simulink model "Regulator_Flow_Sim_1"  (R2022b)
settings: Solver=VariableStepAuto  StartTime=0.0  StopTime=6  RelTol=1e-3
values from neighbouring files (symbols this model uses):
  A_3 = 60*1e-6    (= 6e-05)    [Init_Regulator_Flow_Sim.m]
  Cd_3 = 0.7    [Init_Regulator_Flow_Sim.m]
  Feedforward = 25    [Init_Regulator_Flow_Sim.m]
  gamma_N2 = 1.4    [Init_Regulator_Flow_Sim.m]
  K_v_4 = 0.5    [Init_Regulator_Flow_Sim.m]
  Kv_1_max = 1    [Init_Regulator_Flow_Sim.m]
  Kv_2 = 1    [Init_Regulator_Flow_Sim.m]
  m_1_0 = V_1*rho_1_0    (= 2.59009009009)    [Init_Regulator_Flow_Sim.m]
  m_2_0 = rho_2_0*(V_2-(m_3_0/rho_L))    (= 0.225225225225)    [Init_Regulator_Flow_Sim.m]
  m_3_0 = 8    [Init_Regulator_Flow_Sim.m]
  P_2_0 = P_2_0*1e5    (= 4000000)    [Init_Regulator_Flow_Sim.m]
  P_atm = 0    [Init_Regulator_Flow_Sim.m]
  Pst = 101325    [Init_Regulator_Flow_Sim.m]
  R_N2 = 296    [Init_Regulator_Flow_Sim.m]
  rho_1_0 = (P_1_0)/(R_N2*T_0_N2)    (= 259.009009009)    [Init_Regulator_Flow_Sim.m]
  rho_L = 1000    [Init_Regulator_Flow_Sim.m]
  rhost = Pst/(R_N2*Tst)    (= 1.25320955222)    [Init_Regulator_Flow_Sim.m]
  T_0_N2 = 300    [Init_Regulator_Flow_Sim.m]
  Tst = 273.15    [Init_Regulator_Flow_Sim.m]
  V_1 = V_1*1e-3    (= 0.01)    [Init_Regulator_Flow_Sim.m]
  V_2 = V_2*1e-3    (= 0.013)    [Init_Regulator_Flow_Sim.m]
libraries: slpidlib x2
settings Model: Creator=marti  LastModifiedBy=marti

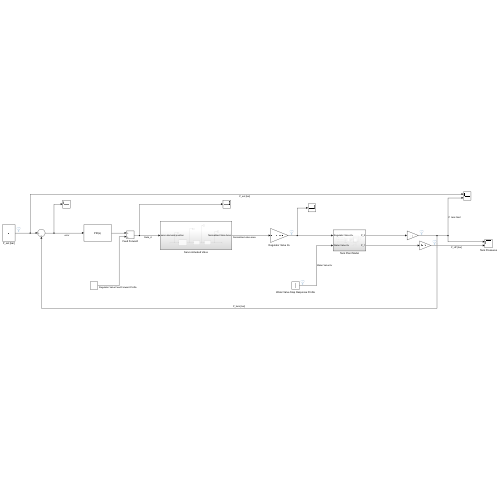
[thumbnail: Simulink's stored preview of the top-level diagram]
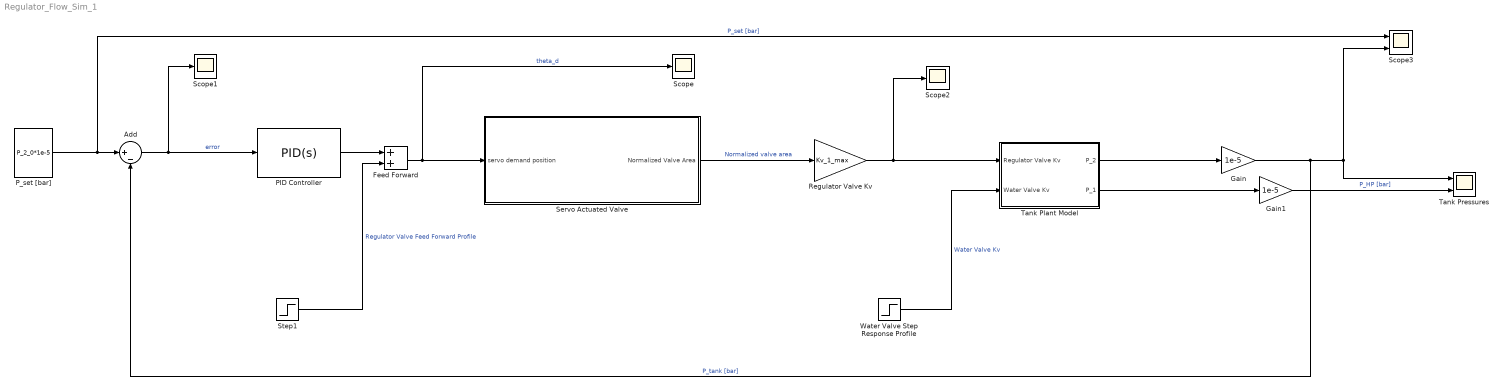
== system Regulator_Flow_Sim_1 ==
  Add : Sum  Inputs=|+-
  Feed Forward : Sum
  Gain : Gain  Gain=1e-5
  Gain1 : Gain  Gain=1e-5
  PID Controller : slpidlib/PID Controller  Controller=PID  Form=Parallel  TimeDomain=Continuous-time  UseExternalTs=off  SampleTime=-1  IntegratorMethod=Forward Euler  FilterMethod=Forward Euler  ControllerParametersSource=internal  P=1.5  I=3  UseKiTs=off  D=0  N=100  UseFilter=on  TunerSelectOption=Transfer Function Based (PID Tuner App)  InitialConditionSource=internal  InitialConditionForIntegrator=0  InitialConditionForFilter=0  DifferentiatorICPrevScaledInput=0  ExternalReset=none  TrackingMode=off  Kt=1  LimitOutput=off  SatLimitsSource=internal  UpperSaturationLimit=180  LowerSaturationLimit=0  LinearizeAsGain=on  AntiWindupMode=clamping  Kb=1  LimitIntegrator=on  UpperIntegratorSaturationLimit=20  LowerIntegratorSaturationLimit=-20  POutMin=[]  POutMax=[]  IOutMin=[]  IOutMax=[]  DOutMin=[]  DOutMax=[]  NOutMin=[]  NOutMax=[]  SumOutMin=[]  SumOutMax=[]  SaturationOutMin=[]  SaturationOutMax=[]  PParamMin=[]  PParamMax=[]  IParamMin=[]  IParamMax=[]  DParamMin=[]  DParamMax=[]  NParamMin=[]  NParamMax=[]  KbParamMin=[]  KbParamMax=[]  KtParamMin=[]  KtParamMax=[]  KbOutMin=[]  KbOutMax=[]  KtOutMin=[]  KtOutMax=[]  IntegratorOutMin=[]  IntegratorOutMax=[]  FilterOutMin=[]  FilterOutMax=[]  SumI1OutMin=[]  SumI1OutMax=[]  SumI2OutMin=[]  SumI2OutMax=[]  SumI3OutMin=[]  SumI3OutMax=[]  SumI4OutMin=[]  SumI4OutMax=[]  SumDOutMin=[]  SumDOutMax=[]  DifferentiatorOutMin=[]  DifferentiatorOutMax=[]  FilterDiffOutCoefMin=[]  FilterDiffOutCoefMax=[]  ReciprocalOutMin=[]  ReciprocalOutMax=[]  SumDenOutMin=[]  SumDenOutMax=[]  SumNumOutMin=[]  SumNumOutMax=[]  DivideOutMin=[]  DivideOutMax=[]  UdiffTsProdOutMin=[]  UdiffTsProdOutMax=[]  NTsProdOutMin=[]  NTsProdOutMax=[]  UintegralTsProdOutMin=[]  UintegralTsProdOutMax=[]  UngainTsProdOutMin=[]  UngainTsProdOutMax=[]  ClampingZeroOutDataTypeStr=Inherit: Inherit via back propagation  ClampingZeroOutMin=[]  ClampingZeroOutMax=[]  FilterDenConstantOutDataTypeStr=Inherit: Inherit via back propagation  FilterDenConstantOutMin=[]  FilterDenConstantOutMax=[]  PCopyOutDataTypeStr=Inherit: Inherit via back propagation  PCopyOutMin=[]  PCopyOutMax=[]  NCopyOutDataTypeStr=Inherit: Inherit via back propagation  NCopyOutMin=[]  NCopyOutMax=[]  IntegratorContinuousStateAttributes=''  IntegratorStateMustResolveToSignalObject=off  IntegratorRTWStateStorageClass=Auto  FilterContinuousStateAttributes=''  FilterStateMustResolveToSignalObject=off  FilterRTWStateStorageClass=Auto  ParallelPVariant=InternalParameters  IdealPVariant=Disabled  IVariant=InternalParameters  DVariant=InternalParameters  IntegratorVariant=Continuous  SatVariant=Disabled  AWVariant=Passthrough  PCopyVariant=Disabled  TRVariant=Disabled  FdbkBlocksVariant=Forward  IdealPFdbkVariant=Disabled  SatFdbkVariant=Disabled  DerivativeFilterVariant=ContFilter  NVariant=InternalParameters  NCopyVariant=Disabled  FilterICVariant=InternalICsFilter  IntegratorICVariant=InternalICs  ExternalResetVariant=Disabled  TRSumVariant=Passthrough  SumFdbkVariant=Disabled  SumVariant=Sum_PID  TsampFilterVariant=InternalTs  TsampNgainVariant=Passthrough  TsampIntegralVariant=Passthrough  ExternalSaturationOutDataTypeStr=Inherit: Same as second input
  P_set [bar] : Constant  Value=P_2_0*1e-5
  Regulator Valve Kv : Gain  Gain=Kv_1_max
  Scope : Scope
  Scope1 : Scope
  Scope2 : Scope
  Scope3 : Scope  NumInputPorts=2
  Servo Actuated Valve : Subsystem
  Step1 : Step  After=Feedforward  SampleTime=0
  Tank Plant Model : Subsystem
  Tank Pressures : Scope  NumInputPorts=2
  Water Valve Step Response Profile : Step  After=Kv_2  SampleTime=0
  wires:
  Water Valve Step Response Profile/1 -> Tank Plant Model/2(Water Valve Kv)  "Water Valve Kv"
  Tank Plant Model/1(P_2) -> Gain/1
  Tank Plant Model/2(P_1) -> Gain1/1
  Servo Actuated Valve/1(Normalized Valve Area) -> Regulator Valve Kv/1  "Normalized valve area"
  Feed Forward/1 -> Scope/1, Servo Actuated Valve/1(servo demand position)  "theta_d"
  Add/1 -> Scope1/1, PID Controller/1  "error"
  Gain/1 -> Scope3/2, Tank Pressures/1, Add/2  "P_tank [bar]"
  Gain1/1 -> Tank Pressures/2  "P_HP [bar]"
  Regulator Valve Kv/1 -> Scope2/1, Tank Plant Model/1(Regulator Valve Kv)
  P_set [bar]/1 -> Scope3/1, Add/1  "P_set [bar]"
  PID Controller/1 -> Feed Forward/1
  Step1/1 -> Feed Forward/2  "Regulator Valve Feed Forward Profile"

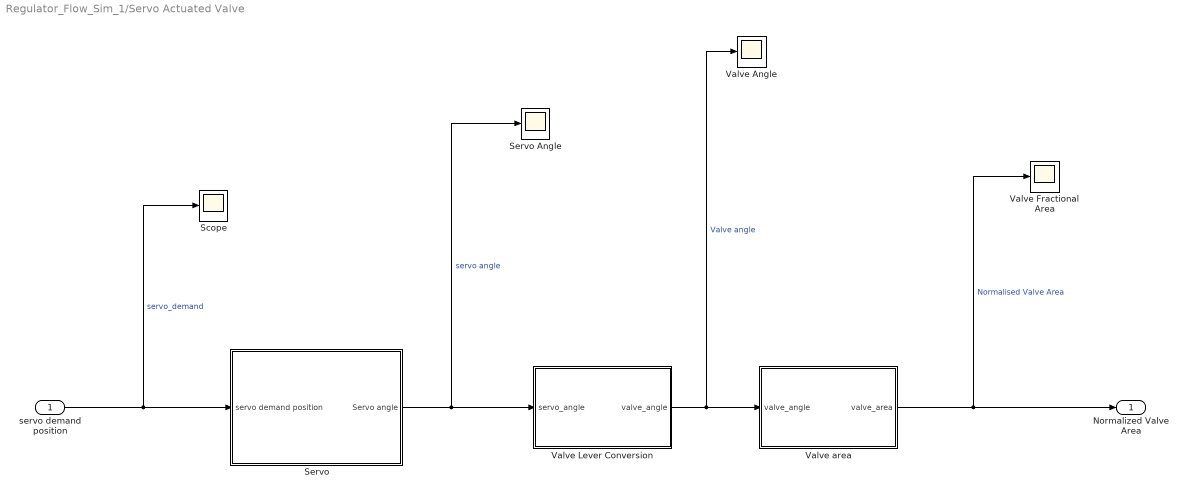
== system Regulator_Flow_Sim_1/Servo Actuated Valve ==
  servo demand position : Inport
  " Valve Lever Conversion" : MATLAB Function  TreatAsAtomicUnit=on
  " Valve area" : MATLAB Function  TreatAsAtomicUnit=on
  Scope : Scope
  Servo : Subsystem
  Servo Angle : Scope
  Valve Angle : Scope
  Valve Fractional Area : Scope
  Normalized Valve Area : Outport
  wires:
  " Valve area"/1(valve_area) -> Normalized Valve Area/1, Valve Fractional Area/1  "Normalised Valve Area"
  " Valve Lever Conversion"/1(valve_angle) -> " Valve area"/1(valve_angle), Valve Angle/1  "Valve angle"
  servo demand position/1 -> Scope/1, Servo/1(servo demand position)  "servo_demand"
  Servo/1(Servo angle) -> " Valve Lever Conversion"/1(servo_angle), Servo Angle/1  "servo angle"

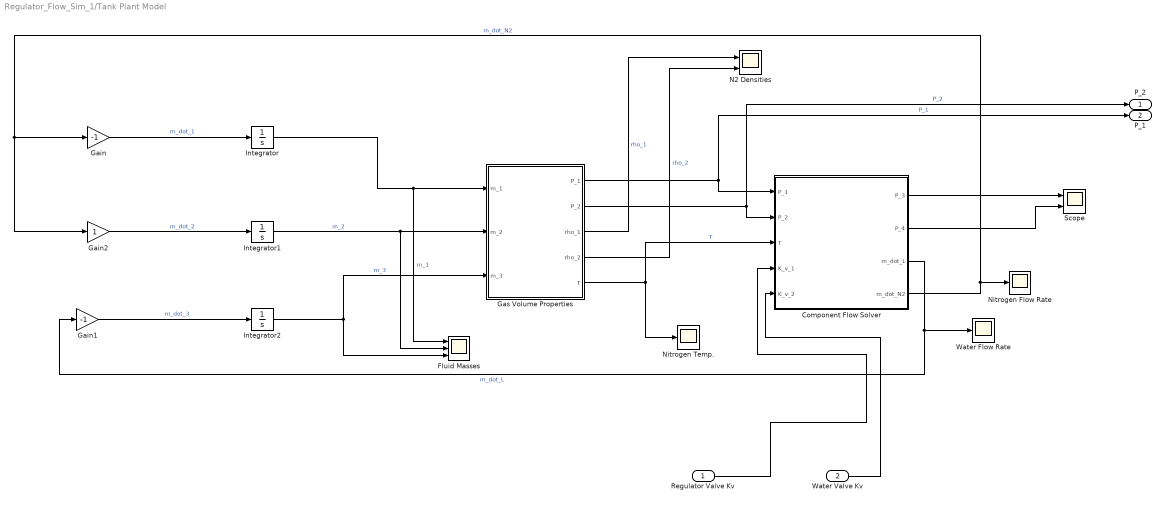
== system Regulator_Flow_Sim_1/Tank Plant Model ==
  Regulator Valve Kv : Inport
  Water Valve Kv : Inport  Port=2
  Component Flow Solver : MATLAB Function  TreatAsAtomicUnit=on
  Fluid Masses : Scope  NumInputPorts=3
  Gain : Gain  Gain=-1
  Gain1 : Gain  Gain=-1
  Gain2 : Gain
  Gas Volume Properties : MATLAB Function  TreatAsAtomicUnit=on
  Integrator : Integrator  InitialCondition=m_1_0
  Integrator1 : Integrator  InitialCondition=m_2_0
  Integrator2 : Integrator  InitialCondition=m_3_0
  N2 Densities : Scope  NumInputPorts=2
  Nitrogen Flow Rate : Scope
  Nitrogen Temp. : Scope
  Scope : Scope  NumInputPorts=2
  Water Flow Rate : Scope
  P_2 : Outport
  P_1 : Outport  Port=2
  wires:
  Gas Volume Properties/1(P_1) -> P_1/1, Component Flow Solver/1(P_1)  "P_1"
  Gain/1 -> Integrator/1  "m_dot_1"
  Component Flow Solver/1(P_3) -> Scope/1
  Integrator1/1 -> Fluid Masses/2, Gas Volume Properties/2(m_2)  "m_2"
  Integrator/1 -> Fluid Masses/1, Gas Volume Properties/1(m_1)  "m_1"
  Component Flow Solver/2(P_4) -> Scope/2
  Gain1/1 -> Integrator2/1  "m_dot_3"
  Component Flow Solver/4(m_dot_N2) -> Nitrogen Flow Rate/1, Gain2/1, Gain/1  "m_dot_N2"
  Gain2/1 -> Integrator1/1  "m_dot_2"
  Integrator2/1 -> Gas Volume Properties/3(m_3), Fluid Masses/3  "m_3"
  Gas Volume Properties/2(P_2) -> P_2/1, Component Flow Solver/2(P_2)  "P_2"
  Component Flow Solver/3(m_dot_L) -> Water Flow Rate/1, Gain1/1  "m_dot_L"
  Gas Volume Properties/4(rho_2) -> N2 Densities/2  "rho_2"
  Gas Volume Properties/3(rho_1) -> N2 Densities/1  "rho_1"
  Gas Volume Properties/5(T) -> Nitrogen Temp./1, Component Flow Solver/3(T)  "T"
  Water Valve Kv/1 -> Component Flow Solver/5(K_v_2)
  Regulator Valve Kv/1 -> Component Flow Solver/4(K_v_1)

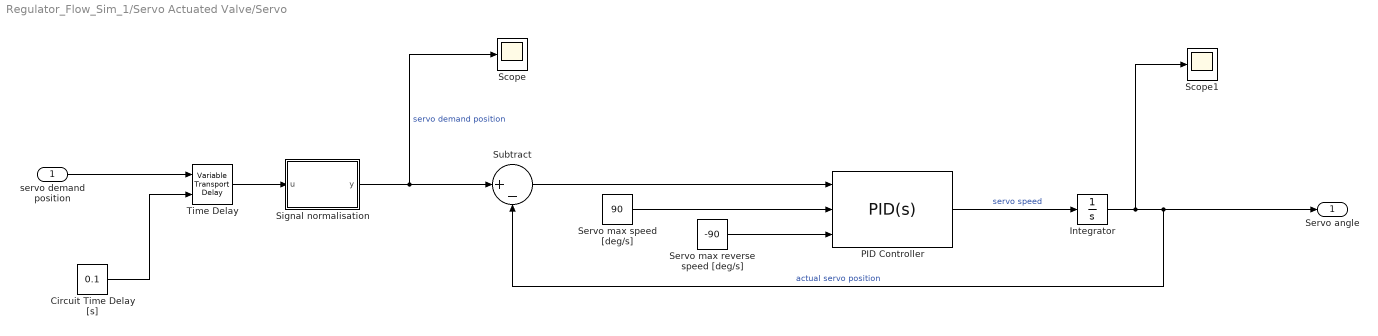
== system Regulator_Flow_Sim_1/Servo Actuated Valve/Servo ==
  servo demand position : Inport
  Circuit Time Delay [s] : Constant  Value=0.1
  Integrator : Integrator
  PID Controller : slpidlib/PID Controller  Controller=PID  Form=Parallel  TimeDomain=Continuous-time  UseExternalTs=off  SampleTime=-1  IntegratorMethod=Forward Euler  FilterMethod=Forward Euler  ControllerParametersSource=internal  P=10  I=1  UseKiTs=off  D=0  N=100  UseFilter=on  TunerSelectOption=Transfer Function Based (PID Tuner App)  InitialConditionSource=internal  InitialConditionForIntegrator=0  InitialConditionForFilter=0  DifferentiatorICPrevScaledInput=0  ExternalReset=none  TrackingMode=off  Kt=1  LimitOutput=on  SatLimitsSource=external  UpperSaturationLimit=inf  LowerSaturationLimit=-inf  LinearizeAsGain=on  AntiWindupMode=none  Kb=1  LimitIntegrator=off  UpperIntegratorSaturationLimit=inf  LowerIntegratorSaturationLimit=-inf  POutMin=[]  POutMax=[]  IOutMin=[]  IOutMax=[]  DOutMin=[]  DOutMax=[]  NOutMin=[]  NOutMax=[]  SumOutMin=[]  SumOutMax=[]  SaturationOutMin=[]  SaturationOutMax=[]  PParamMin=[]  PParamMax=[]  IParamMin=[]  IParamMax=[]  DParamMin=[]  DParamMax=[]  NParamMin=[]  NParamMax=[]  KbParamMin=[]  KbParamMax=[]  KtParamMin=[]  KtParamMax=[]  KbOutMin=[]  KbOutMax=[]  KtOutMin=[]  KtOutMax=[]  IntegratorOutMin=[]  IntegratorOutMax=[]  FilterOutMin=[]  FilterOutMax=[]  SumI1OutMin=[]  SumI1OutMax=[]  SumI2OutMin=[]  SumI2OutMax=[]  SumI3OutMin=[]  SumI3OutMax=[]  SumI4OutMin=[]  SumI4OutMax=[]  SumDOutMin=[]  SumDOutMax=[]  DifferentiatorOutMin=[]  DifferentiatorOutMax=[]  FilterDiffOutCoefMin=[]  FilterDiffOutCoefMax=[]  ReciprocalOutMin=[]  ReciprocalOutMax=[]  SumDenOutMin=[]  SumDenOutMax=[]  SumNumOutMin=[]  SumNumOutMax=[]  DivideOutMin=[]  DivideOutMax=[]  UdiffTsProdOutMin=[]  UdiffTsProdOutMax=[]  NTsProdOutMin=[]  NTsProdOutMax=[]  UintegralTsProdOutMin=[]  UintegralTsProdOutMax=[]  UngainTsProdOutMin=[]  UngainTsProdOutMax=[]  ClampingZeroOutDataTypeStr=Inherit: Inherit via back propagation  ClampingZeroOutMin=[]  ClampingZeroOutMax=[]  FilterDenConstantOutDataTypeStr=Inherit: Inherit via back propagation  FilterDenConstantOutMin=[]  FilterDenConstantOutMax=[]  PCopyOutDataTypeStr=Inherit: Inherit via back propagation  PCopyOutMin=[]  PCopyOutMax=[]  NCopyOutDataTypeStr=Inherit: Inherit via back propagation  NCopyOutMin=[]  NCopyOutMax=[]  IntegratorContinuousStateAttributes=''  IntegratorStateMustResolveToSignalObject=off  IntegratorRTWStateStorageClass=Auto  FilterContinuousStateAttributes=''  FilterStateMustResolveToSignalObject=off  FilterRTWStateStorageClass=Auto  ParallelPVariant=InternalParameters  IdealPVariant=Disabled  IVariant=InternalParameters  DVariant=InternalParameters  IntegratorVariant=Continuous  SatVariant=External  AWVariant=Passthrough  PCopyVariant=Disabled  TRVariant=Disabled  FdbkBlocksVariant=Forward  IdealPFdbkVariant=Disabled  SatFdbkVariant=Disabled  DerivativeFilterVariant=ContFilter  NVariant=InternalParameters  NCopyVariant=Disabled  FilterICVariant=InternalICsFilter  IntegratorICVariant=InternalICs  ExternalResetVariant=Disabled  TRSumVariant=Passthrough  SumFdbkVariant=Disabled  SumVariant=Sum_PID  TsampFilterVariant=InternalTs  TsampNgainVariant=Passthrough  TsampIntegralVariant=Passthrough  ExternalSaturationOutDataTypeStr=Inherit: Same as second input
  Scope : Scope
  Scope1 : Scope
  Servo max reverse speed [deg/s] : Constant  Value=-90
  Servo max speed [deg/s] : Constant  Value=90
  Signal normalisation : MATLAB Function  TreatAsAtomicUnit=on
  Subtract : Sum  Inputs=|+-
  Time Delay : VariableTransportDelay  MaximumDelay=10
  Servo angle : Outport
  wires:
  Servo max reverse speed [deg/s]/1 -> PID Controller/3
  Servo max speed [deg/s]/1 -> PID Controller/2
  PID Controller/1 -> Integrator/1  "servo speed"
  Integrator/1 -> Scope1/1, Servo angle/1, Subtract/2  "actual servo position"
  Subtract/1 -> PID Controller/1
  Signal normalisation/1(y) -> Scope/1, Subtract/1  "servo demand position"
  servo demand position/1 -> Time Delay/1
  Time Delay/1 -> Signal normalisation/1(u)
  Circuit Time Delay [s]/1 -> Time Delay/2

== matlab function Regulator_Flow_Sim_1/Tank Plant Model/Component Flow Solver ==
  data: P_1 input; P_2 input; P_3 output; T input; P_4 output; m_dot_L output; m_dot_N2 output; K_v_1 input; K_v_2 input; Cd_3 parameter; K_v_4 parameter; rho_L parameter; R_N2 parameter; Tst parameter; rhost parameter; P_atm parameter; A_3 parameter; Pst parameter
function [P_3,P_4,m_dot_L,m_dot_N2]= fcn(P_1,P_2,T,K_v_1,K_v_2,Cd_3,K_v_4,rho_L,R_N2,Tst,rhost,P_atm,A_3, Pst)

P_1 = P_1*1e-5;
P_2 = P_2*1e-5;

fun = @(x)paramfun(x,P_1,P_2,T,K_v_1,K_v_2,A_3,Cd_3,K_v_4,rho_L,R_N2,Pst,Tst,rhost,P_atm); %Define set of non-linear equations to rootfind on
x0 = [1,1,1,1]; %Define initial guesses
options = optimoptions('fsolve','Algorithm','levenberg-marquardt');
x = fsolve(fun,x0,options); %Solve system of equations 

P_3 = x(1)*1e5;
P_4 = x(2)*1e5;
m_dot_L = x(3);
m_dot_N2 = x(4);

function F = paramfun(x,P_1,P_2,T,K_v_1,K_v_2,A_3,Cd_3,K_v_4,rho_L,R_N2,Pst,Tst,rhost,P_atm)
P_3 = x(1);
P_4 = x(2);
m_dot_L = x(3);
m_dot_N2 = x(4);

%Regulator Valve
if (P_4 >= 0.528*P_1)
    %non-choked flow
    Q_N = K_v_1*514*(((P_1-P_4)*P_4)/(rhost*T))/sqrt(abs(((P_1-P_4)*P_4)/(rhost*T)));
else
    %choked flow
    Q_N = K_v_1*257*P_1/sqrt(abs(rhost*T));
end
m_dot_c = Q_N*(Pst/(R_N2*Tst))*(1/3600); %Convert standard flow rate to mass flow rate

%Check Valve (K_v_4)
if (P_2 >= 0.528*P_4)
    %non-choked flow
    Q_N = K_v_4*514*(((P_4-P_2)*P_2)/(rhost*T))/sqrt(abs(((P_4-P_2)*P_2)/(rhost*T)));
else
    %choked flow
    Q_N = K_v_4*257*P_4/sqrt(abs(rhost*T));
end
m_dot_d = Q_N*(Pst/(R_N2*Tst))*(1/3600); %Convert standard flow rate to mass flow rate

%Water Control Valve
SG = rho_L/1000; %Calculate specific gravity of propellant (value for water is 1)
Q = K_v_2*((P_2 - P_3)/SG)/sqrt(abs((P_2 - P_3)/SG)); %Calculate volumetric flow rate based on Kv
m_dot_a = Q*rho_L*(1/3600); %Convert standard flow rate to mass flow rate

%Water Orifice
m_dot_b = Cd_3*A_3*2*rho_L*(P_3*1e5 - P_atm)/sqrt(abs(2*rho_L*(P_3*1e5 - P_atm)));

F = [m_dot_L - m_dot_a, m_dot_L - m_dot_b, m_dot_N2 - m_dot_c, m_dot_N2 - m_dot_d];

== matlab function Regulator_Flow_Sim_1/Tank Plant Model/Gas Volume Properties ==
  data: P_1 output; P_2 output; m_1 input; rho_1 output; m_2 input; m_3 input; rho_2 output; T output; V_1 parameter; V_2 parameter; T_0_N2 parameter; rho_1_0 parameter; gamma_N2 parameter; R_N2 parameter; rho_L parameter
function [P_1, P_2, rho_1, rho_2, T]= fcn(m_1, m_2, m_3, V_1, V_2, T_0_N2, rho_1_0, gamma_N2, R_N2, rho_L)

rho_1 = m_1/V_1; %Find the HP tank gas density
rho_2 = m_2/(V_2 - m_3/rho_L); %Find the ullage gas density
T = T_0_N2*(rho_1/rho_1_0)^(gamma_N2 - 1); %Find the ullage gas temperature (assumiong adiabatic expansion)
P_1 = rho_1*R_N2*T; %Find the HP gas pressure
P_2 = rho_2*R_N2*T; %Find the ullage gas pressure (Tank pressure)

== matlab function Regulator_Flow_Sim_1/Servo Actuated Valve/ Valve Lever Conversion ==
  data: servo_angle input; valve_angle output
function valve_angle = fcn(servo_angle)

theta = deg2rad(servo_angle - 20);

% Define lengths of the different levers
g = 42; %Distance between pivots [mm]
a = 20; %Servo Horn Length [mm]
b = 38; %Valve Lever Length [mm]
h = 61; %Connecting linkage length [mm]

fun = @(x)paramfun(x,theta,g,a,b,h); %Define set of non-linear equations to rootfind on
x0 = [pi/2,pi]; %Define initial guesses
options = optimoptions('fsolve','Algorithm','levenberg-marquardt');
x = fsolve(fun,x0,options); %Solve system of equations 

psi = x(2);

valve_angle = rad2deg(psi) - 66;

% Function used for iteratively solving the 
function F = paramfun(x, theta,g,a,b,h)
phi = x(1);
psi = x(2);
F = [a*cos(theta) - h*cos(phi) - b*cos(psi) + g, a*sin(theta) + h*sin(phi) - b*sin(psi)];

== matlab function Regulator_Flow_Sim_1/Servo Actuated Valve/ Valve area ==
  data: valve_angle input; valve_area output
function valve_area = fcn(valve_angle)
valve_angle = valve_angle - 5; %Account for first part of rotation where valve doesn't open at all
if valve_angle < 0
    valve_area = 0;
else
    valve_area = 1.1*((5*10^-6)*valve_angle^3 - 0.0006*valve_angle^2 + 0.0278*valve_angle); %calculate normalised valve area
end

== matlab function Regulator_Flow_Sim_1/Servo Actuated Valve/Servo/Signal normalisation ==
  data: u input; y output
function y = fcn(u)
if u < 0
    y = 0;
else 
    if u > 180
        y = 180;
    else
        y = u;
    end
end
